simulink model "simple_model"  (R2019a)
settings: Solver=VariableStepDiscrete  StartTime=0.0  StopTime=10  MaxStep=2  RelTol=1e-3
libraries: simulink x1
settings Model: EnablePacing=on  Creator=wuyuanyi  LastModifiedBy=wuyuanyi

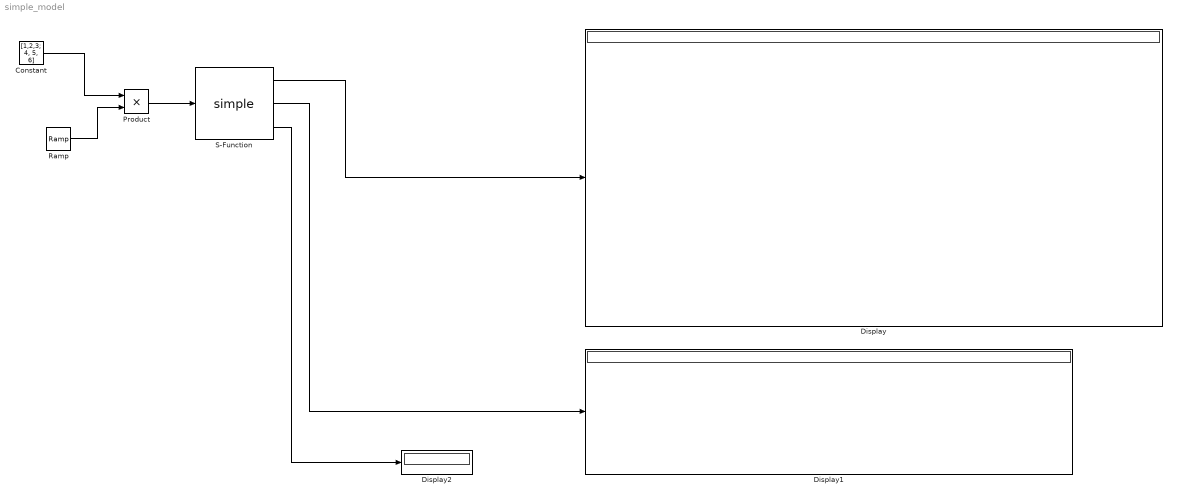
== system simple_model ==
  Constant : Constant  Value=[1,2,3; 4, 5, 6]
  Display : Display
  Display1 : Display
  Display2 : Display
  Product : Product
  Ramp : simulink/Sources/Ramp  slope=1  start=0  InitialOutput=0
  S-Function : S-Function  FunctionName=simple  SFunctionDeploymentMode=off  EnableBusSupport=off
  wires:
  S-Function/1 -> Display/1
  S-Function/2 -> Display1/1
  S-Function/3 -> Display2/1
  Constant/1 -> Product/1
  Product/1 -> S-Function/1
  Ramp/1 -> Product/2
